simulink model "simulink_pendulum"  (R2025a)
settings: Solver=VariableStepAuto  StartTime=0.0  StopTime=15  RelTol=1e-3
model workspace: external: MAT-File (data not in the file)
values from neighbouring files (symbols this model uses):
  a = [m*l^2; beta; m*g*l]    [setvar_pendulum.m]
  A = [0 1 0 ... (first row only)    [setvar_pendulum.m]
  a_hat_0 = 10*a    [setvar_pendulum.m]
  B = [0; 0; k^3]    [setvar_pendulum.m]
  beta = 0.05    [setvar_pendulum.m]
  C = [1 0 0 ... (first row only)    [setvar_pendulum.m]
  D = [0; 0; 0]    [setvar_pendulum.m]
  g = 9.81    [setvar_pendulum.m]
  Gamma = diag([1,10,10])    [setvar_pendulum.m]
  Gamma_discrete = diag([1,10,10])*h_Adapt    [setvar_pendulum.m]
  h_Adapt = 0.0001    [setvar_pendulum.m]
  Kd = m*l^2 * 20    (= 0.04)    [setvar_pendulum.m]
  l = 0.1    [PendulumAnimation.m]    (also in setvar_pendulum.m)
  lambda = Kp/Kd    (= 150)    [setvar_pendulum.m]
  m = 0.2    [setvar_pendulum.m]
  noise_power = (0.1* pi/180)^2    (= 3.04617419787e-06)    [setvar_pendulum.m]
  q_0 = 20 * pi/180    (= 0.349065850399)    [setvar_pendulum.m]
  qd = 0 * pi/180    (= 0)    [setvar_pendulum.m]
  qd_0 = [q_0; 0; 0]    [setvar_pendulum.m]
  qd_freq_rad = 2*pi*f    (= 4.18879020479)    [setvar_pendulum.m]
  qdot_0 = 50 * pi/180    (= 0.872664625997)    [setvar_pendulum.m]
  sigma = 0.1    [setvar_pendulum.m]
libraries: simulink x2
settings Model: Creator=olesd  LastModifiedBy=olesd

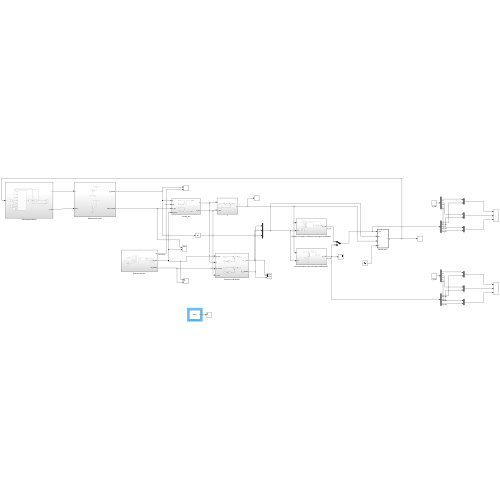
[thumbnail: Simulink's stored preview of the top-level diagram]
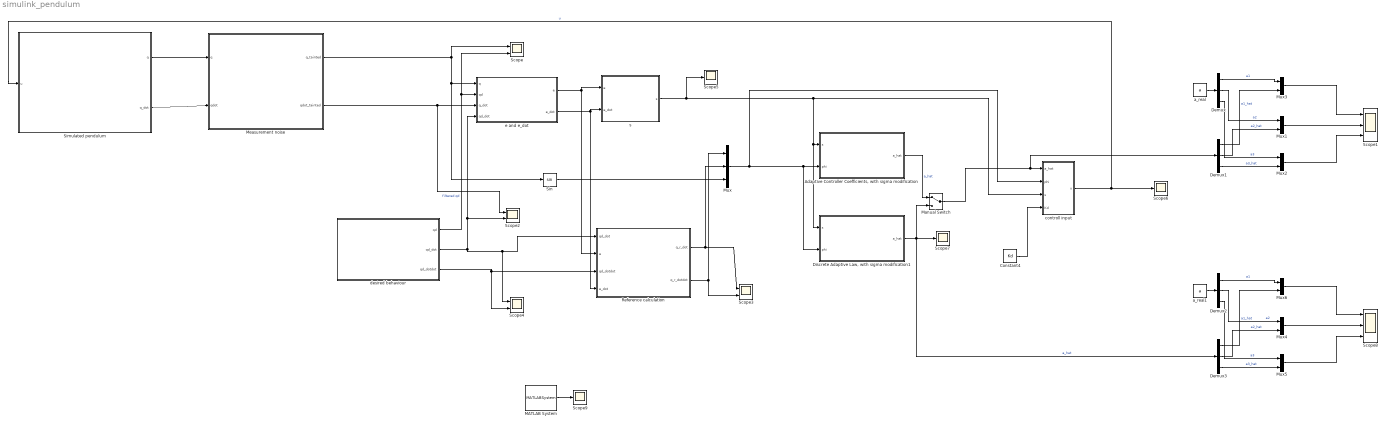
== system simulink_pendulum ==
  "Adaptive Controller Coefficients, with sigma modification" : Subsystem
  Constant4 : Constant  Value=Kd
  Demux{,1..3} (4 alike) : Demux  Outputs=3
  "Discrete Adaptive Law, with sigma modification1" : Subsystem
  MATLAB System : MATLABSystem  System=test1  SimulateUsing=Interpreted execution
      mask Type: test1
  Manual Switch : ManualSwitch
  Measurement noise : Subsystem
  Mux : Mux  Inputs=3
  Mux{1..6} (6 alike) : Mux  Inputs=2
  Reference calculation : Subsystem
  Scope{,2..4} (4 alike) : Scope  NumInputPorts=2
      Scope settings: ActiveDisplayYMinimum=-1.3223485512123507  ActiveDisplayYMaximum=1.3311085005564014
      Scope2 settings: ActiveDisplayYMinimum=-0.233112357060524  ActiveDisplayYMaximum=2.0969862516059683  DataLoggingVariableName=ScopeData8
      Scope3 settings: ActiveDisplayYMinimum=-150.23287759936176  ActiveDisplayYMaximum=40.147404968405745  DataLoggingVariableName=ScopeData3
      Scope4 settings: ActiveDisplayYMinimum=-2.0040208560030712  ActiveDisplayYMaximum=18.036187704027647  DataLoggingVariableName=ScopeData4
  Scope1 : Scope  NumInputPorts=3
      settings: ActiveDisplayString=3  ActiveDisplayYMinimum=-0.5879994906904592  ActiveDisplayYMaximum=2.2453332767433851
  Scope{5..7,9} (4 alike) : Scope
      Scope5 settings: ActiveDisplayYMinimum=0.21309211831446717  ActiveDisplayYMaximum=3.6522263444102858  DataLoggingVariableName=ScopeData5
      Scope6 settings: ActiveDisplayYMinimum=-22.426996970374024  ActiveDisplayYMaximum=-22.426906344016569  DataLoggingVariableName=ScopeData6
      Scope7 settings: ActiveDisplayYMinimum=-2.8025507650856283  ActiveDisplayYMaximum=1.6283910937645658  DataLoggingVariableName=ScopeData9
      Scope9 settings: ActiveDisplayYMinimum=-2.8777191571351315  ActiveDisplayYMaximum=15.262870412025865  DataLoggingVariableName=ScopeData11
  Scope8 : Scope  NumInputPorts=3
      settings: ActiveDisplayString=3  ActiveDisplayYMinimum=-0.024522542471835135  ActiveDisplayYMaximum=2.1827028822465171  DataLoggingVariableName=ScopeData10
  Simulated pendulum : Subsystem
  Sin : Trigonometry
  a_real : Constant  Value=a  VectorParams1D=off  SampleTime=-1
  a_real1 : Constant  Value=a  VectorParams1D=off  SampleTime=-1
  controll input : MATLAB Function  TreatAsAtomicUnit=on
  desired behaviour : Subsystem
  e and e_dot : Subsystem
  s : Subsystem
  wires:
  e and e_dot/1(e) -> s/1(e), Reference calculation/2(e)
  e and e_dot/2(e_dot) -> s/2(e_dot), Reference calculation/4(e_dot)
  desired behaviour/1(qd) -> Scope/2, e and e_dot/2(qd)  "filtered qd"
  desired behaviour/2(qd_dot) -> Scope4/1, Reference calculation/1(qd_dot), Scope2/2, e and e_dot/4(qd_dot)
  desired behaviour/3(qd_dotdot) -> Scope4/2, Reference calculation/3(qd_dotdot)
  Reference calculation/2(q_r_dotdot) -> Scope3/2, Mux/1
  Reference calculation/1(q_r_dot) -> Scope3/1, Mux/2
  Mux/1 -> "Discrete Adaptive Law, with sigma modification1"/2(phi), "Adaptive Controller Coefficients, with sigma modification"/2(phi), controll input/2(phi)
  s/1(s) -> controll input/3(s), "Discrete Adaptive Law, with sigma modification1"/1(s), "Adaptive Controller Coefficients, with sigma modification"/1(s), Scope5/1
  Constant4/1 -> controll input/4(Kd)
  Sin/1 -> Mux/3
  a_real/1 -> Demux/1
  Demux/2 -> Mux1/1  "a2"
  Demux1/2 -> Mux1/2  "a2_hat"
  Demux1/3 -> Mux2/2  "a3_hat"
  Demux/3 -> Mux2/1  "a3"
  Demux/1 -> Mux3/1  "a1"
  Demux1/1 -> Mux3/2  "a1_hat"
  Mux1/1 -> Scope1/2
  Mux3/1 -> Scope1/1
  Mux2/1 -> Scope1/3
  controll input/1(u) -> Simulated pendulum/1(u), Scope6/1  "u"
  Simulated pendulum/1(q) -> Measurement noise/1(q)
  Simulated pendulum/2(q_dot) -> Measurement noise/2(qdot)
  Measurement noise/1(q_tainted) -> Sin/1, e and e_dot/1(q), Scope/1
  Measurement noise/2(qdot_tainted) -> Scope2/1, e and e_dot/3(q_dot)
  "Adaptive Controller Coefficients, with sigma modification"/1(a_hat) -> Manual Switch/1  "a_hat"
  "Discrete Adaptive Law, with sigma modification1"/1(a_hat) -> Demux3/1, Scope7/1, Manual Switch/2  "a_hat"
  Manual Switch/1 -> Demux1/1, controll input/1(a_hat)
  Mux4/1 -> Scope8/2
  Demux3/1 -> Mux6/2  "a1_hat"
  Mux6/1 -> Scope8/1
  Demux2/1 -> Mux6/1  "a1"
  Demux2/3 -> Mux5/1  "a3"
  Demux3/2 -> Mux4/2  "a2_hat"
  a_real1/1 -> Demux2/1
  Mux5/1 -> Scope8/3
  Demux2/2 -> Mux4/1  "a2"
  Demux3/3 -> Mux5/2  "a3_hat"
  MATLAB System/1 -> Scope9/1

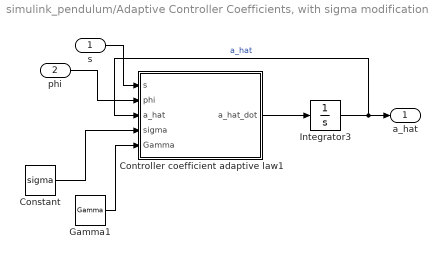
== system simulink_pendulum/Adaptive Controller Coefficients, with sigma modification ==
  s : Inport
  phi : Inport  Port=2
  Constant : Constant  Value=sigma
  Controller coefficient adaptive law1 : MATLAB Function  TreatAsAtomicUnit=on
  Gamma1 : Constant  Value=Gamma
  Integrator3 : Integrator  InitialCondition=a_hat_0
  a_hat : Outport
  wires:
  Controller coefficient adaptive law1/1(a_hat_dot) -> Integrator3/1
  s/1 -> Controller coefficient adaptive law1/1(s)
  phi/1 -> Controller coefficient adaptive law1/2(phi)
  Gamma1/1 -> Controller coefficient adaptive law1/5(Gamma)
  Integrator3/1 -> Controller coefficient adaptive law1/3(a_hat), a_hat/1  "a_hat"
  Constant/1 -> Controller coefficient adaptive law1/4(sigma)

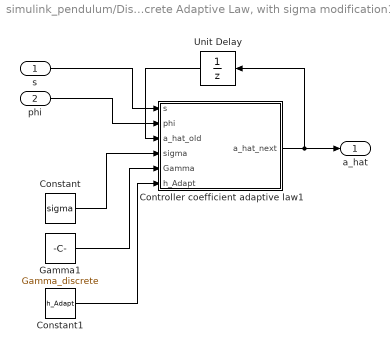
== system simulink_pendulum/Discrete Adaptive Law, with sigma modification1 ==
  s : Inport
  phi : Inport  Port=2
  Constant : Constant  Value=sigma
  Constant1 : Constant  Value=h_Adapt
  Controller coefficient adaptive law1 : MATLAB Function  TreatAsAtomicUnit=on  SystemSampleTime=h_Adapt
  Gamma1 : Constant  Value=Gamma_discrete
  Unit Delay : UnitDelay  InitialCondition=a_hat_0  SampleTime=h_Adapt  HasFrameUpgradeWarning=on
  a_hat : Outport
  wires:
  s/1 -> Controller coefficient adaptive law1/1(s)
  phi/1 -> Controller coefficient adaptive law1/2(phi)
  Gamma1/1 -> Controller coefficient adaptive law1/5(Gamma)
  Constant/1 -> Controller coefficient adaptive law1/4(sigma)
  Controller coefficient adaptive law1/1(a_hat_next) -> Unit Delay/1, a_hat/1
  Constant1/1 -> Controller coefficient adaptive law1/6(h_Adapt)
  Unit Delay/1 -> Controller coefficient adaptive law1/3(a_hat_old)

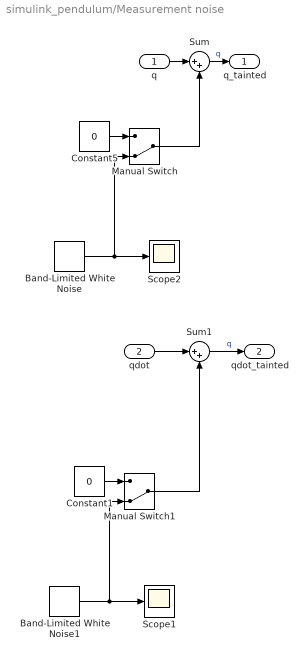
== system simulink_pendulum/Measurement noise ==
  q : Inport
  qdot : Inport  Port=2
  Band-Limited White Noise : simulink/Sources/Band-Limited White Noise  Cov=[noise_power]  Ts=0.1  seed=[23341]
  Band-Limited White Noise1 : simulink/Sources/Band-Limited White Noise  Cov=[noise_power]  Ts=0.1  seed=[23341]
  Constant1 : Constant  Value=0
  Constant5 : Constant  Value=0
  Manual Switch : ManualSwitch  CurrentSetting=0
  Manual Switch1 : ManualSwitch  CurrentSetting=0
  Scope1 : Scope
      settings: ActiveDisplayYMinimum=-1  ActiveDisplayYMaximum=1  DataLoggingVariableName=ScopeData7
  Scope2 : Scope
      settings: ActiveDisplayYMinimum=-1  ActiveDisplayYMaximum=1  DataLoggingVariableName=ScopeData2
  Sum : Sum  Inputs=|++
  Sum1 : Sum  Inputs=|++
  q_tainted : Outport
  qdot_tainted : Outport  Port=2
  wires:
  Constant5/1 -> Manual Switch/1
  Manual Switch/1 -> Sum/2
  Sum/1 -> q_tainted/1  "q"
  q/1 -> Sum/1
  Band-Limited White Noise/1 -> Manual Switch/2, Scope2/1
  Constant1/1 -> Manual Switch1/1
  Manual Switch1/1 -> Sum1/2
  Band-Limited White Noise1/1 -> Manual Switch1/2, Scope1/1
  qdot/1 -> Sum1/1
  Sum1/1 -> qdot_tainted/1  "q"

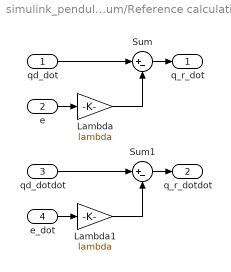
== system simulink_pendulum/Reference calculation ==
  qd_dot : Inport
  e : Inport  Port=2
  qd_dotdot : Inport  Port=3
  e_dot : Inport  Port=4
  Lambda : Gain  Gain=lambda
  Lambda1 : Gain  Gain=lambda
  Sum : Sum  Inputs=|+-
  Sum1 : Sum  Inputs=|+-
  q_r_dot : Outport
  q_r_dotdot : Outport  Port=2
  wires:
  qd_dot/1 -> Sum/1
  e/1 -> Lambda/1
  Sum/1 -> q_r_dot/1
  Lambda1/1 -> Sum1/2
  Lambda/1 -> Sum/2
  qd_dotdot/1 -> Sum1/1
  e_dot/1 -> Lambda1/1
  Sum1/1 -> q_r_dotdot/1

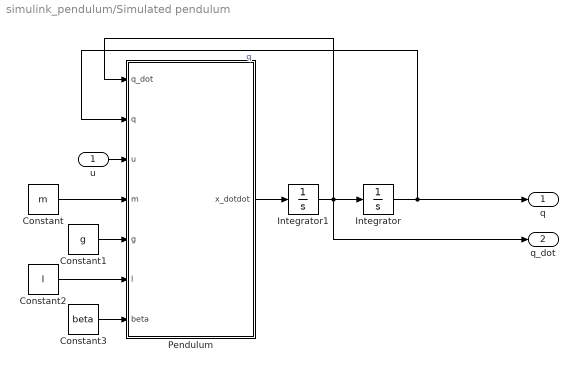
== system simulink_pendulum/Simulated pendulum ==
  u : Inport
  Constant : Constant  Value=m
  Constant1 : Constant  Value=g
  Constant2 : Constant  Value=l
  Constant3 : Constant  Value=beta
  Integrator : Integrator  InitialCondition=q_0
  Integrator1 : Integrator  InitialCondition=qdot_0
  Pendulum : MATLAB Function  TreatAsAtomicUnit=on
  q : Outport
  q_dot : Outport  Port=2
  wires:
  Integrator/1 -> q/1, Pendulum/2(q)  "q"
  u/1 -> Pendulum/3(u)
  Constant3/1 -> Pendulum/7(beta)
  Integrator1/1 -> q_dot/1, Integrator/1, Pendulum/1(q_dot)
  Constant/1 -> Pendulum/4(m)
  Constant1/1 -> Pendulum/5(g)
  Constant2/1 -> Pendulum/6(l)
  Pendulum/1(x_dotdot) -> Integrator1/1

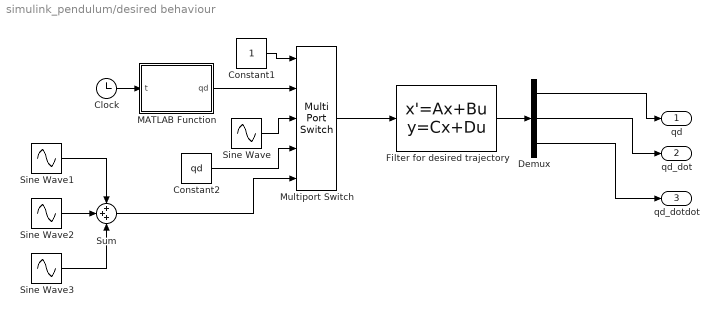
== system simulink_pendulum/desired behaviour ==
  Clock : Clock
  Constant1 : Constant
  Constant2 : Constant  Value=qd
  Demux : Demux  Outputs=3
  Filter for desired trajectory : StateSpace  A=A  B=B  C=C  D=D  InitialCondition=qd_0
  MATLAB Function : MATLAB Function  TreatAsAtomicUnit=on
  Multiport Switch : MultiPortSwitch  Inputs=4  SaturateOnIntegerOverflow=off  InputSameDT=off
  Sine Wave : Sin  Amplitude=0.2  Frequency=qd_freq_rad  SampleTime=0
  Sine Wave1 : Sin  Frequency=qd_freq_rad  SampleTime=0
  Sine Wave2 : Sin  Amplitude=0.05  Frequency=qd_freq_rad*10  SampleTime=0
  Sine Wave3 : Sin  Amplitude=0.05  Frequency=qd_freq_rad*0.01  SampleTime=0
  Sum : Sum  Inputs=+++
  qd : Outport
  qd_dot : Outport  Port=2
  qd_dotdot : Outport  Port=3
  wires:
  Constant1/1 -> Multiport Switch/1
  Multiport Switch/1 -> Filter for desired trajectory/1
  Sine Wave/1 -> Multiport Switch/3
  Constant2/1 -> Multiport Switch/4
  Sine Wave2/1 -> Sum/2
  Sine Wave1/1 -> Sum/1
  Sine Wave3/1 -> Sum/3
  Sum/1 -> Multiport Switch/5
  Filter for desired trajectory/1 -> Demux/1
  Demux/1 -> qd/1
  Demux/2 -> qd_dot/1
  Demux/3 -> qd_dotdot/1
  Clock/1 -> MATLAB Function/1(t)
  MATLAB Function/1(qd) -> Multiport Switch/2

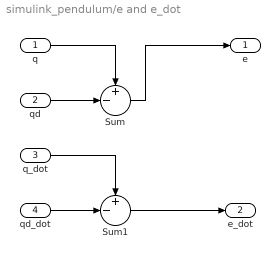
== system simulink_pendulum/e and e_dot ==
  q : Inport
  qd : Inport  Port=2
  q_dot : Inport  Port=3
  qd_dot : Inport  Port=4
  Sum : Sum  Inputs=+-|
  Sum1 : Sum  Inputs=+-|
  e : Outport
  e_dot : Outport  Port=2
  wires:
  Sum/1 -> e/1
  q/1 -> Sum/1
  Sum1/1 -> e_dot/1
  qd/1 -> Sum/2
  qd_dot/1 -> Sum1/2
  q_dot/1 -> Sum1/1

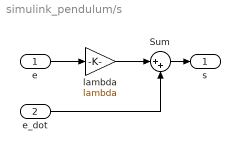
== system simulink_pendulum/s ==
  e : Inport
  e_dot : Inport  Port=2
  Sum : Sum  Inputs=|++
  lambda : Gain  Gain=lambda
  s : Outport
  wires:
  Sum/1 -> s/1
  e/1 -> lambda/1
  lambda/1 -> Sum/1
  e_dot/1 -> Sum/2

== matlab function simulink_pendulum/Discrete Adaptive Law, with sigma modification1/Controller coefficient adaptive law1 ==
  data: s input; phi input; a_hat_old input; sigma input; Gamma input; a_hat_next output; h_Adapt input
function a_hat_next = fcn(s, phi, a_hat_old, sigma, Gamma, h_Adapt)
    a_hat_next = a_hat_old + h_Adapt*(-Gamma*s*phi- sigma*a_hat_old);
end

== matlab function simulink_pendulum/Simulated pendulum/Pendulum ==
  data: q_dot input size=1; q input size=1; u input; x_dotdot output; m input; g input; l input; beta input
function x_dotdot  = fcn(q_dot, q, u, m, g, l, beta)
    x_dotdot = 1/(m*l^2) * (u - m*g*l*sin(q) - beta*q_dot);
end

== matlab function simulink_pendulum/controll input ==
  data: a_hat input; u output; phi input; s input; Kd input
function u = fcn(a_hat, phi, s, Kd)
u = a_hat' * phi - Kd*s;

== matlab function simulink_pendulum/desired behaviour/MATLAB Function ==
  data: t input; qd output
function qd = fcn(t)
    if 0 <= t && t <= 3
        qd = 60* pi/180;
    elseif 3 < t && t <= 6
        qd = -60 * pi/180;
    else
        qd = 0;
    end

== matlab function simulink_pendulum/Adaptive Controller Coefficients, with sigma modification/Controller coefficient adaptive law1 ==
  data: s input; phi input; a_hat input; sigma input; Gamma input; a_hat_dot output
function a_hat_dot = fcn(s, phi, a_hat, sigma, Gamma)
    a_hat_dot = -Gamma*s*phi - sigma*a_hat;
    
end
